simulink model "a23_kreis"  (R2014a)
settings: Solver=ode45  StartTime=0.0  StopTime=10.0  RelTol=1e-3
settings Model: Creator=s65556  LastModifiedBy=s65556

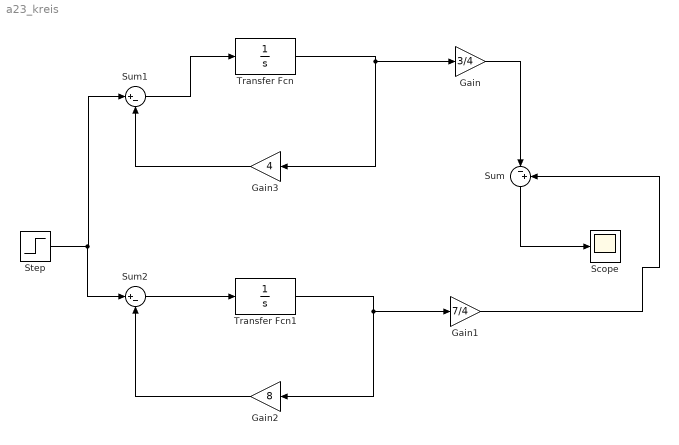
== system a23_kreis ==
  Gain : Gain  Gain=3/4
  Gain1 : Gain  Gain=7/4
  Gain2 : Gain  Gain=8
  Gain3 : Gain  Gain=4
  Scope : Scope
  Step : Step  SampleTime=0
  Sum : Sum  Inputs=|-+
  Sum1 : Sum  Inputs=|+-
  Sum2 : Sum  Inputs=|+-
  Transfer Fcn : TransferFcn  Denominator=[1 0]
  Transfer Fcn1 : TransferFcn  Denominator=[1 0]
  wires:
  Step/1 -> Sum2/1, Sum1/1
  Sum1/1 -> Transfer Fcn/1
  Transfer Fcn/1 -> Gain3/1, Gain/1
  Gain3/1 -> Sum1/2
  Transfer Fcn1/1 -> Gain2/1, Gain1/1
  Gain2/1 -> Sum2/2
  Sum2/1 -> Transfer Fcn1/1
  Gain1/1 -> Sum/2
  Gain/1 -> Sum/1
  Sum/1 -> Scope/1
